simulink model "mpc_model"  (Simulink 7.0)
settings: Solver=ode45  StartTime=0.0  StopTime=Tsim-Ts  RelTol=1e-3
values from neighbouring files (symbols this model uses):
  pcd = c2d(pc, Ts, 'zoh')    [date_init.m]
settings Model: Creator=B014  LastModifiedBy=B014

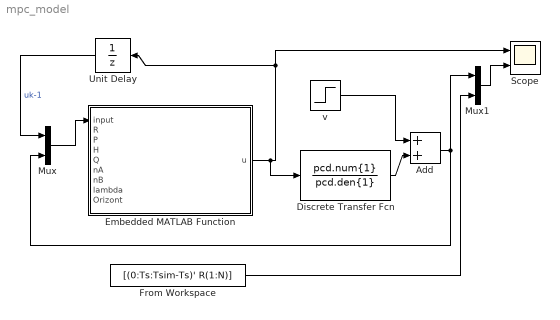
== system mpc_model ==
  Add : Sum  OutDataType=sfix(16)  OutScaling=2^-10
  Discrete Transfer Fcn : DiscreteTransferFcn  Numerator=pcd.num{1}  Denominator=pcd.den{1}
  Embedded MATLAB Function : Stateflow chart
  From Workspace : FromWorkspace  VariableName=[(0:Ts:Tsim-Ts)' R(1:N)]  SampleTime=0
  Mux : Mux  Inputs=2
  Mux1 : Mux  Inputs=2
  Scope : Scope  NumInputPorts=2
      settings: YMin=-5~-5  YMax=5~5
  Unit Delay : UnitDelay  Orientation=left
  v : Step  SampleTime=0
  wires:
  Unit Delay/1 -> Mux/1  "uk-1"
  Mux/1 -> Embedded MATLAB Function/1(input)
  Discrete Transfer Fcn/1 -> Add/2
  v/1 -> Add/1
  From Workspace/1 -> Mux1/2
  Add/1 -> Mux1/1, Mux/2
  Embedded MATLAB Function/1(u) -> Scope/1, Unit Delay/1, Discrete Transfer Fcn/1
  Mux1/1 -> Scope/2

== matlab function Embedded MATLAB Function ==
  data: input input inherited; u output inherited; R input inherited; P input inherited; H input inherited; Q input inherited; nA input inherited; nB input inherited; lambda input inherited; Orizont input inherited
function u = myMPC(input,R,P,H,Q,nA,nB,lambda,Orizont)
persistent yPast uPast k

if isempty(yPast)
    yPast=zeros(2, 1);
    uPast=zeros(1, 1);
    k = 1;
end

for i = length(uPast):-1:2
    uPast(i)=uPast(i-1);
end
uPast(1)=input(1);
for i=length(yPast):-1:2
    yPast(i)=yPast(i-1);
end
yPast(1)=input(2);

Rs=[R(k+1) R(k+1) R(k+1)]';
Sol = -inv(P'*Q*P + lambda*eye(3)) * P * Q * (H * [yPast;uPast] - Rs);
u = Sol(1);

k = k+1;

end
